simulink model "sldvdemo_sbr_verification_fixed_replacement"  (R2021b)
settings: Solver=FixedStepDiscrete  StartTime=0.0  StopTime=10.0  FixedStep=0.01  RelTol=1e-3  EnableMultiTasking=on
PreLoadFcn:
  | load sldvdemo_sbrBusDef
model workspace (MAT data in the model file):
  BLINK_TIME = Simulink.Parameter
  BLINK_TIME.Value = 5
  BLINK_TIME.DataType = 'uint16'
  BLINK_TIME.Complexity = 'real'
  BLINK_TIME.Dimensions = [1 1]
  SPEED_LIMIT = embedded.fi
  SPEED_LIMIT.DataType = 'Fixed'
  SPEED_LIMIT.Scaling = 'BinaryPoint'
  SPEED_LIMIT.Signed = 0
  SPEED_LIMIT.WordLength = 16
  SPEED_LIMIT.FixedExponent = -2
  SPEED_LIMIT.SlopeAdjustmentFactor = 1
  SPEED_LIMIT.Bias = 0
  SPEED_LIMIT.DataTypeOverride = 'Inherit'
  SPEED_LIMIT.intarray = 60
  SPEED_LIMIT.noverflows = 0
  SPEED_LIMIT.nunderflows = 0
  SPEED_LIMIT.maxlog = -1.79769313486e+308
  SPEED_LIMIT.minlog = 1.79769313486e+308
  SPEED_LIMIT.RoundingMethod = 'Nearest'
  SPEED_LIMIT.OverflowAction = 'Saturate'
  SPEED_LIMIT.ProductMode = 'FullPrecision'
  SPEED_LIMIT.SumMode = 'FullPrecision'
  SPEED_LIMIT.ProductWordLength = 32
  SPEED_LIMIT.SumWordLength = 32
  SPEED_LIMIT.MaxProductWordLength = 65535
  SPEED_LIMIT.MaxSumWordLength = 65535
  SPEED_LIMIT.ProductFractionLength = 30
  SPEED_LIMIT.ProductFixedExponent = -30
  SPEED_LIMIT.ProductSlope = 9.31322574615e-10
  SPEED_LIMIT.ProductSlopeAdjustmentFactor = 1
  SPEED_LIMIT.ProductBias = 0
  SPEED_LIMIT.SumFractionLength = 30
  SPEED_LIMIT.SumFixedExponent = -30
  SPEED_LIMIT.SumSlope = 9.31322574615e-10
  SPEED_LIMIT.SumSlopeAdjustmentFactor = 1
  SPEED_LIMIT.SumBias = 0
  SPEED_LIMIT.CastBeforeSum = 1
  SPEED_LIMIT.DDGMaxProductWordLength = 65535
  SPEED_LIMIT.DDGMaxSumWordLength = 65535
  SPEED_LIMIT.DDGProductFixedExponent = -30
  SPEED_LIMIT.DDGProductFractionLength = 30
  SPEED_LIMIT.DDGProductWordLength = 32
  SPEED_LIMIT.DDGSumFixedExponent = -30
  SPEED_LIMIT.DDGSumFractionLength = 30
  SPEED_LIMIT.DDGSumWordLength = 32
  SPEED_LIMIT.DDGCastBeforeSum = 1
  SPEED_LIMIT.DDGProductBias = 0
  SPEED_LIMIT.DDGProductSlopeAdjustmentFactor = 1
  SPEED_LIMIT.DDGSumBias = 0
  SPEED_LIMIT.DDGSumSlopeAdjustmentFactor = 1
  SPEED_LIMIT.DDGProductSlope = 9.31322574615e-10
  SPEED_LIMIT.DDGSumSlope = 9.31322574615e-10
  SPEED_LIMIT.Logging = 0
  SPEED_LIMIT.fimathislocal = 0
undefined symbols (not defined in the file or in its folder): sldvsubsys
libraries: sldvlib x4
Description:
  | Property Proving Using MATLAB Function Block
settings Model: DVDesignModelName=sldvdemo_sbr_verification_fixed  Creator=The MathWorks, Inc.  LastModifiedBy=Alessandro
settings SolverCC: AlgebraicLoopSolver=TrustRegion
settings DataIOCC: ExternalInput=testdata  LimitDataPoints=on  SaveFormat=Array  ReturnWorkspaceOutputs=off
settings OptimizationCC: ExpressionDepthLimit=2147483647  InitFltsAndDblsToZero=on  LifeSpan=1  EfficientTunableParamExpr=on
settings DebuggingCC: UnderspecifiedInitializationDetection=Classic  MergeDetectMultiDrivingBlocksExec=none  SolverPrmCheckMsg=warning  FcnCallInpInsideContextMsg=warning  AllowSymbolicDim=off  StateNameClashWarn=warning  SymbolicDimsDataTypeCodeGenerationDiagnostic=none  SFUnexpectedBacktrackingDiag=warning  SFNoUnconditionalDefaultTransitionDiag=warning  SFExecutionAtInitializationDiag=none  SFMachineParentedDataDiag=warning  ArithmeticOperatorsInVariantConditions=warning
settings HardwareCC: ProdBitPerPointer=32  ProdBitPerSizeT=32  ProdBitPerPtrDiffT=32  ProdLargestAtomicFloat=None  ProdIntDivRoundTo=Undefined  ProdEndianess=Unspecified  ProdWordSize=32  ProdHWDeviceType=32-bit Generic
settings ModelReferenceCC: PropagateSignalLabelsOutOfModel=off
settings SFSimCC: SimUseLocalCustomCode=off  SimParseCustomCode=off  MATLABDynamicMemAlloc=off  CustomCodeUndefinedFunction=UseInterfaceOnly
settings RTWCC: Description=Real-Time Workshop Embedded Coder (no auto configuration)  SystemTargetFile=ert.tlc  GenCodeOnly=on  TemplateMakefile=ert_default_tmf  RTWUseLocalCustomCode=off
settings CodeAppCC: IgnoreCustomStorageClasses=off  CustomSymbolStrType=$N$R$M  CustomSymbolStrModelFcn=$N  StateflowObjectComments=on  InternalIdentifier=Classic
settings ERTTargetCC: MultiwordLength=2048  GenerateSampleERTMain=on  ERTCustomFileTemplate=example_file_process.tlc  ConvertIfToSwitch=off  SuppressUnreachableDefaultCases=off
settings ConfigComp: DVMode=PropertyProving  DVMaxProcessTime=600  DVParameters=on  DVModelCoverageObjectives=MCDC  DVMaxTestCaseSteps=500  DVTestSuiteOptimization=Auto  DVDetectActiveLogic=on  DVSaveReport=on  DVRebuildModelRepresentation=Always

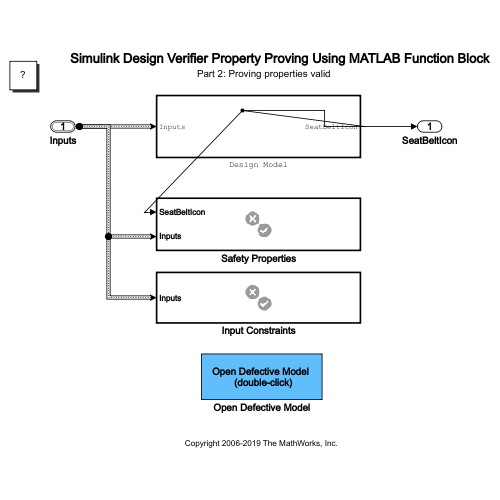
[thumbnail: Simulink's stored preview of the top-level diagram]
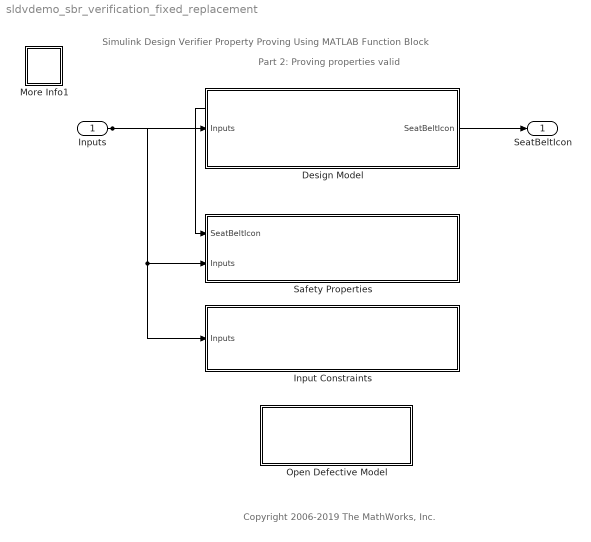
== system sldvdemo_sbr_verification_fixed_replacement ==
  note: Simulink Design Verifier Property Proving Using MATLAB Function Block
  note: Copyright 2006-2019 The MathWorks, Inc.
  note: Part 2: Proving properties valid
  Inputs : Inport  OutDataTypeStr=Bus: sbrInputs  BusOutputAsStruct=on
  Design Model : Subsystem  TreatAsAtomicUnit=on  mask(Sldv ModelReference(Model name:sldvdemo_sbr_design) Replacement){ModelName=sldvdemo_sbr_design, ParameterArgumentNames=, ParameterArgumentValuesAsString=, SimulationMode=Normal}
      mask help: Replacement for the Model Reference block that references the model sldvdemo_sbr_design. If Model arguments are specified on the Model Reference block, then they will appear in the mask parameters.
  Input Constraints : Subsystem  Tag=VerificationSubsystem  DisableCoverage=on  LoadFcn=sldvsubsys('check')  TreatAsAtomicUnit=on  SimViewingDevice=on  mask(VerificationSubsystem){}
      mask init:
      | sldvsubsys('maskInit');
      settings: CopyFcn=sldvsubsys('copy');  OpenFcn=open_system(gcb,'force');
      settings: PreSaveFcn=|
      | set_param(gcb,'SimViewingDevice','on');
      | sldvsubsys('check');
      mask Help: helpview(fullfile(docroot,'toolbox','sldv','sldv.map'),'verificationsubsystem')
      mask Display: image(imread('sldvicon_versubsys.png','BackGroundColor',[1 1 1]),'center');
  More Info1 : Subsystem
      settings: OpenFcn=showExample('sldv/PropertyProvingMATLABFunctionBlockExample')
      mask Display: disp('?')
  Open Defective Model : Subsystem
      settings: OpenFcn=open_system('sldvdemo_sbr_verification');
      mask Display: disp('Open Defective Model \n (double-click)')
  Safety Properties : Subsystem  Tag=VerificationSubsystem  DisableCoverage=on  LoadFcn=sldvsubsys('check')  TreatAsAtomicUnit=on  SimViewingDevice=on  mask(VerificationSubsystem){}
      mask init:
      | sldvsubsys('maskInit');
      settings: CopyFcn=sldvsubsys('copy');  OpenFcn=open_system(gcb,'force');
      settings: PreSaveFcn=|
      | set_param(gcb,'SimViewingDevice','on');
      | sldvsubsys('check');
      mask Help: helpview(fullfile(docroot,'toolbox','sldv','sldv.map'),'verificationsubsystem')
      mask Display: image(imread('sldvicon_versubsys.png','BackGroundColor',[1 1 1]),'center');
  SeatBeltIcon : Outport  OutDataTypeStr=boolean  PortDimensions=1  VectorParamsAs1DForOutWhenUnconnected=off
  wires:
  Inputs/1 -> Design Model/1(Inputs), Safety Properties/2(Inputs), Input Constraints/1(Inputs)
  Design Model/1(SeatBeltIcon) -> SeatBeltIcon/1, Safety Properties/1(SeatBeltIcon)

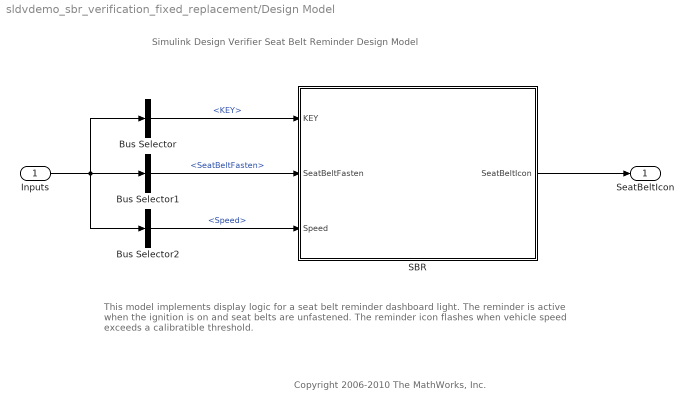
== system sldvdemo_sbr_verification_fixed_replacement/Design Model ==
  note: This model implements display logic for a seat belt reminder dashboard light.  The reminder is active
      | when the ignition is on and seat belts are unfastened.  The reminder icon flashes when vehicle speed
      | exceeds a calibratible threshold.
  note: Copyright 2006-2010 The MathWorks, Inc.
  note: Simulink Design Verifier Seat Belt Reminder Design Model
  Inputs : Inport  OutDataTypeStr=Bus: sbrInputs  SampleTime=[0.01,0]  BusOutputAsStruct=on
  Bus Selector : BusSelector  OutputSignals=KEY
  Bus Selector1 : BusSelector  OutputSignals=SeatBeltFasten
  Bus Selector2 : BusSelector  OutputSignals=Speed
  SBR : Stateflow chart  TreatAsAtomicUnit=on
  SeatBeltIcon : Outport  OutDataTypeStr=boolean  PortDimensions=1  SampleTime=[0.01,0]  VectorParamsAs1DForOutWhenUnconnected=off
  wires:
  Inputs/1 -> Bus Selector1/1, Bus Selector/1, Bus Selector2/1
  Bus Selector2/1 -> SBR/3(Speed)  "<Speed>"
  Bus Selector1/1 -> SBR/2(SeatBeltFasten)  "<SeatBeltFasten>"
  Bus Selector/1 -> SBR/1(KEY)  "<KEY>"
  SBR/1(SeatBeltIcon) -> SeatBeltIcon/1

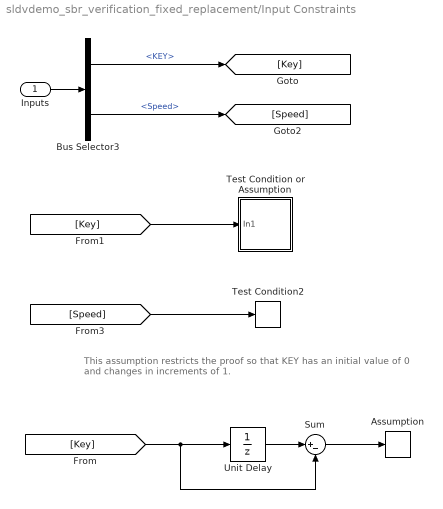
== system sldvdemo_sbr_verification_fixed_replacement/Input Constraints ==
  note: This assumption restricts the proof so that KEY has an
      | initial value of 0 and changes in increments of 1.
  Inputs : Inport
  Assumption : sldvlib/Objectives and Constraints/Assumption  enabled=on  customAVTBlockType=Assumption  intervals=int8([-1 1])  initial=off  dispValues=on  outEnabled=off
      settings: AttributesFormatString=%<intervals>  SourceProductBaseCode=SL
  Bus Selector3 : BusSelector  OutputSignals=KEY,Speed
  Sum : Sum  Inputs=|+-
  Test Condition or Assumption : Subsystem  mask(Design Verifier Test Condition or Assumption){intervals={int8(0),int8(1),int8(2)}}
      mask prompts: intervals "Values"
      mask help: Includes Design Verifier Assumption and Design Verifier Test Condition blocks that are connected to the same input. The block behaves as a Test Condition block in test generation, and as an Assumption block for property proving.
      settings: AttributesFormatString=%<intervals>
      mask Display:
      | image(imread('sldvicon_a_normal.png','BackGroundColor',[1 1 1]),[24 4 21 20]); hide_arrows(true);
      | image(imread('sldvicon_c_normal.png','BackGroundColor',[1 1 1]),[4 24 20 21]); hide_arrows(true);
  Test Condition2 : sldvlib/Objectives and Constraints/Test Condition  enabled=on  customAVTBlockType=Test Condition  intervals=fi([10 30],fixdt(0,16,2))  initial=off  dispValues=on  outEnabled=off
      settings: AttributesFormatString=%<intervals>  SourceProductBaseCode=SL
  Unit Delay : UnitDelay  SampleTime=-1  HasFrameUpgradeWarning=on
  wires:
  Inputs/1 -> Bus Selector3/1
  Bus Selector3/1 -> [Key]  "<KEY>"
  Bus Selector3/2 -> [Speed]  "<Speed>"
  [Key] -> Test Condition or Assumption/1(In1)
  [Speed] -> Test Condition2/1
  Unit Delay/1 -> Sum/1
  Sum/1 -> Assumption/1
  [Key] -> Sum/2, Unit Delay/1

== system sldvdemo_sbr_verification_fixed_replacement/More Info1 ==

== system sldvdemo_sbr_verification_fixed_replacement/Open Defective Model ==

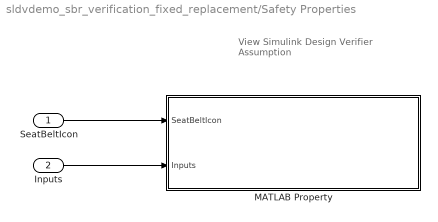
== system sldvdemo_sbr_verification_fixed_replacement/Safety Properties ==
  note: View Simulink Design Verifier
      | Assumption
  SeatBeltIcon : Inport
  Inputs : Inport  Port=2
  MATLAB Property : MATLAB Function  TreatAsAtomicUnit=on
  wires:
  Inputs/1 -> MATLAB Property/2(Inputs)
  SeatBeltIcon/1 -> MATLAB Property/1(SeatBeltIcon)

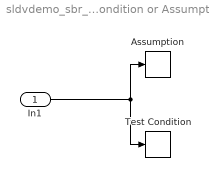
== system sldvdemo_sbr_verification_fixed_replacement/Input Constraints/Test Condition or Assumption ==
  In1 : Inport
  Assumption : sldvlib/Objectives and Constraints/Assumption  enabled=on  customAVTBlockType=Assumption  intervals=intervals  initial=off  dispValues=on  outEnabled=off
      settings: AttributesFormatString=%<intervals>  SourceProductBaseCode=SL
  Test Condition : sldvlib/Objectives and Constraints/Test Condition  enabled=on  customAVTBlockType=Test Condition  intervals=intervals  initial=off  dispValues=on  outEnabled=off
      settings: AttributesFormatString=%<intervals>  SourceProductBaseCode=SL
  wires:
  In1/1 -> Test Condition/1, Assumption/1

== stateflow chart sldvdemo_sbr_verification_fixed_replacement/Design Model/SBR ==
  settings: executeAtInitialization=1
  state Note [group]
    note: This design assumes that the KEY
        | input is initially 0.
  state KEY_CRANK
    entry: SeatBeltIcon=1;
  state KEY_OFF
    entry: SeatBeltIcon=0;
  state KEY_ON
    state SB_UNFASTEN
      state LOW_SPEED
        entry: SeatBeltIcon = 1;
      state HIGH_SPEED
        state OFF
          entry: SeatBeltIcon=0;
        state ON
          entry: SeatBeltIcon=1;
        (default) -> OFF
        OFF -> ON : [after(BLINK_TIME,tick)]
        ON -> OFF : [after(BLINK_TIME,tick)]
      (default) -> LOW_SPEED
      LOW_SPEED -> HIGH_SPEED : [Speed > SPEED_LIMIT]
      HIGH_SPEED -> LOW_SPEED : [Speed <= SPEED_LIMIT]
    state SB_FASTEN
      en: SeatBeltIcon=0;
    (default) -> (junction 26)
    (junction 26) -> SB_UNFASTEN [order 2]
    (junction 26) -> SB_FASTEN [order 1] : [SeatBeltFasten == 1]
    SB_UNFASTEN -> SB_FASTEN : [SeatBeltFasten == 1]
    SB_FASTEN -> SB_UNFASTEN : [SeatBeltFasten == 0]
  (default) -> KEY_OFF
  KEY_OFF -> KEY_ON : [KEY == 1]
  KEY_ON -> KEY_OFF [order 1] : [KEY == 0]
  KEY_ON -> KEY_CRANK [order 2] : [KEY == 2]
  KEY_CRANK -> KEY_ON : [KEY == 1]
  data: KEY input; SeatBeltIcon output boolean; SeatBeltFasten input; Speed input; BLINK_TIME parameter; SPEED_LIMIT parameter fixdt(0,16,2)

== matlab function sldvdemo_sbr_verification_fixed_replacement/Safety Properties/MATLAB Property ==
  data: SeatBeltIcon input boolean; Inputs input sbrInputs
function check_reminder(SeatBeltIcon,Inputs) %#codegen
    % The seat belt light should be active whenever the key is turned on
    % and speed is less than 15 and the seatbelt is not fastened
    activeCond = ((Inputs.KEY ~= 0) && (Inputs.SeatBeltFasten == 0) && ...
                  (Inputs.Speed < 15));
              
    sldv.prove(implies(activeCond,SeatBeltIcon));

function out = implies(cond, result)
    if (cond)
        out = result;
    else
        out = true;
    end
